simulink model "k1visbs"  (Simulink 8.6)
settings: Solver=ode45  StartTime=0.0  StopTime=10.0  RelTol=1e-3
libraries: cdsEpicsOut x10, cdsBit2Word x10, cdsFilt x8, cdsEpicsBinIn x5, cdsWord2Bit x5, cdsCDI64 x5, cdsCDO64 x5, dac x2, cdsAdcx0 x1, cdsAdcx1 x1, TYPEB_MASTER x1, cdsIPCx x1
(part 1 of 2)
settings Model: Creator=controls  LastModifiedBy=controls
settings DataIOCC: SignalLoggingSaveFormat=Dataset
settings OptimizationCC: ExpressionDepthLimit=128
settings DebuggingCC: UnderspecifiedInitializationDetection=Simplified  MergeDetectMultiDrivingBlocksExec=error  SolverPrmCheckMsg=none  FcnCallInpInsideContextMsg=EnableAllAsError  StateNameClashWarn=none
settings GRTTargetCC: CombineOutputUpdateFcns=on  GRTInterface=off

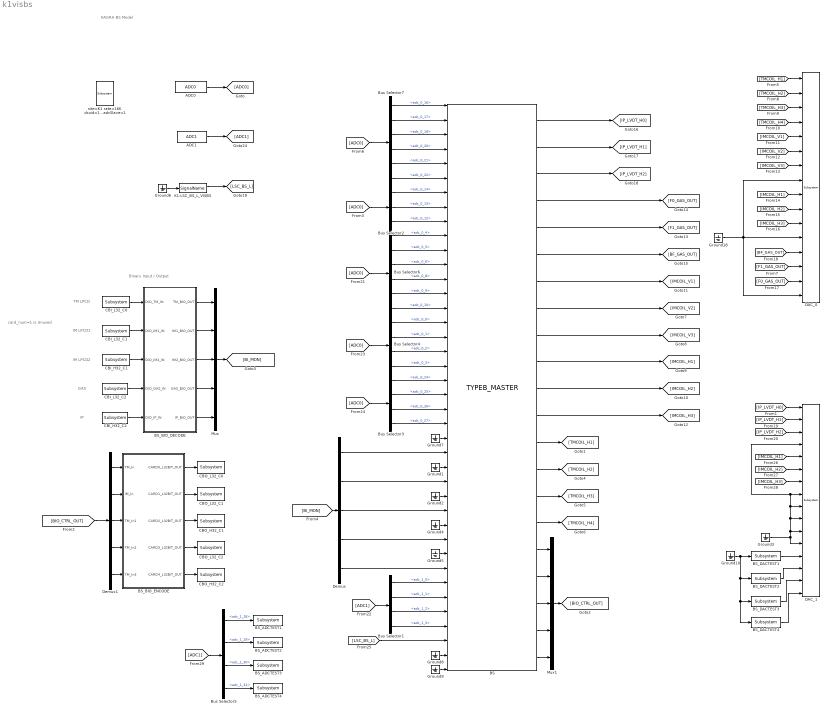
== system k1visbs ==
  note: TM LPCD
  note: KAGRA BS Model
  note: Binary Input / Output
  note: card_num=1 is Unused
  note: IM LPCD1
  note: IM LPCD2
  note: GAS
  note: IP
  ADC0 : cdsAdcx0/ADC0  Tag=cdsAdc  Description=|
      | type-GSC_16AI64SSA
      | card_num=0
      settings: AttributesFormatString=%<Description>\n%<Tag>
  ADC1 : cdsAdcx1/ADC1  Tag=cdsAdc  Description=|
      | type-GSC_16AI64SSA
      | card_num=1
      settings: AttributesFormatString=%<Description>\n%<Tag>
  BS : TYPEB_MASTER/TYPEB_MASTER
  BS_ADCTEST1 : cdsFilt/Subsystem  Tag=cdsFilt  Description=|
      | Purpose:                                                                                                                                                                                                                                  
      | Standard CDS IIR filter module.                                                                                                                                                                                                           
      |                                                                                                                                                                                                                                           
      | Operation:                                                                                                                                                                                                                                
      | Consists of 10 second order section IIR filters, plus a ramped gain stage. In FE code, also provides pre-defined test points and excitation channel inputs. The filter coefficients are defined in the LIGO system using the 'foton' tool.
      |                                                                                                                                                                                                                                           
      | Usage:                                                                                                                                                                                                                                    
      | Name the part with the desired filter module name.
      settings: AttributesFormatString=%<Tag>
  BS_ADCTEST2 : cdsFilt/Subsystem  Tag=cdsFilt  Description=|
      | Purpose:                                                                                                                                                                                                                                  
      | Standard CDS IIR filter module.                                                                                                                                                                                                           
      |                                                                                                                                                                                                                                           
      | Operation:                                                                                                                                                                                                                                
      | Consists of 10 second order section IIR filters, plus a ramped gain stage. In FE code, also provides pre-defined test points and excitation channel inputs. The filter coefficients are defined in the LIGO system using the 'foton' tool.
      |                                                                                                                                                                                                                                           
      | Usage:                                                                                                                                                                                                                                    
      | Name the part with the desired filter module name.
      settings: AttributesFormatString=%<Tag>
  BS_ADCTEST3 : cdsFilt/Subsystem  Tag=cdsFilt  Description=|
      | Purpose:                                                                                                                                                                                                                                  
      | Standard CDS IIR filter module.                                                                                                                                                                                                           
      |                                                                                                                                                                                                                                           
      | Operation:                                                                                                                                                                                                                                
      | Consists of 10 second order section IIR filters, plus a ramped gain stage. In FE code, also provides pre-defined test points and excitation channel inputs. The filter coefficients are defined in the LIGO system using the 'foton' tool.
      |                                                                                                                                                                                                                                           
      | Usage:                                                                                                                                                                                                                                    
      | Name the part with the desired filter module name.
      settings: AttributesFormatString=%<Tag>
  BS_ADCTEST4 : cdsFilt/Subsystem  Tag=cdsFilt  Description=|
      | Purpose:                                                                                                                                                                                                                                  
      | Standard CDS IIR filter module.                                                                                                                                                                                                           
      |                                                                                                                                                                                                                                           
      | Operation:                                                                                                                                                                                                                                
      | Consists of 10 second order section IIR filters, plus a ramped gain stage. In FE code, also provides pre-defined test points and excitation channel inputs. The filter coefficients are defined in the LIGO system using the 'foton' tool.
      |                                                                                                                                                                                                                                           
      | Usage:                                                                                                                                                                                                                                    
      | Name the part with the desired filter module name.
      settings: AttributesFormatString=%<Tag>
  BS_BIO_DECODE : Subsystem
  BS_BIO_ENCODE : Subsystem
  BS_DACTEST1 : cdsFilt/Subsystem  Tag=cdsFilt  Description=|
      | Purpose:                                                                                                                                                                                                                                  
      | Standard CDS IIR filter module.                                                                                                                                                                                                           
      |                                                                                                                                                                                                                                           
      | Operation:                                                                                                                                                                                                                                
      | Consists of 10 second order section IIR filters, plus a ramped gain stage. In FE code, also provides pre-defined test points and excitation channel inputs. The filter coefficients are defined in the LIGO system using the 'foton' tool.
      |                                                                                                                                                                                                                                           
      | Usage:                                                                                                                                                                                                                                    
      | Name the part with the desired filter module name.
      settings: AttributesFormatString=%<Tag>
  BS_DACTEST2 : cdsFilt/Subsystem  Tag=cdsFilt  Description=|
      | Purpose:                                                                                                                                                                                                                                  
      | Standard CDS IIR filter module.                                                                                                                                                                                                           
      |                                                                                                                                                                                                                                           
      | Operation:                                                                                                                                                                                                                                
      | Consists of 10 second order section IIR filters, plus a ramped gain stage. In FE code, also provides pre-defined test points and excitation channel inputs. The filter coefficients are defined in the LIGO system using the 'foton' tool.
      |                                                                                                                                                                                                                                           
      | Usage:                                                                                                                                                                                                                                    
      | Name the part with the desired filter module name.
      settings: AttributesFormatString=%<Tag>
  BS_DACTEST3 : cdsFilt/Subsystem  Tag=cdsFilt  Description=|
      | Purpose:                                                                                                                                                                                                                                  
      | Standard CDS IIR filter module.                                                                                                                                                                                                           
      |                                                                                                                                                                                                                                           
      | Operation:                                                                                                                                                                                                                                
      | Consists of 10 second order section IIR filters, plus a ramped gain stage. In FE code, also provides pre-defined test points and excitation channel inputs. The filter coefficients are defined in the LIGO system using the 'foton' tool.
      |                                                                                                                                                                                                                                           
      | Usage:                                                                                                                                                                                                                                    
      | Name the part with the desired filter module name.
      settings: AttributesFormatString=%<Tag>
  BS_DACTEST4 : cdsFilt/Subsystem  Tag=cdsFilt  Description=|
      | Purpose:                                                                                                                                                                                                                                  
      | Standard CDS IIR filter module.                                                                                                                                                                                                           
      |                                                                                                                                                                                                                                           
      | Operation:                                                                                                                                                                                                                                
      | Consists of 10 second order section IIR filters, plus a ramped gain stage. In FE code, also provides pre-defined test points and excitation channel inputs. The filter coefficients are defined in the LIGO system using the 'foton' tool.
      |                                                                                                                                                                                                                                           
      | Usage:                                                                                                                                                                                                                                    
      | Name the part with the desired filter module name.
      settings: AttributesFormatString=%<Tag>
  Bus Selector1 : BusSelector  Description=ADC Selector  OutputSignals=adc_1_0,adc_1_1,adc_1_2,adc_1_3
      settings: AttributesFormatString=%<Description>
  Bus Selector2 : BusSelector  Description=ADC Selector  OutputSignals=adc_0_14,adc_0_13,adc_0_12
      settings: AttributesFormatString=%<Description>
  Bus Selector3 : BusSelector  Description=ADC Selector  OutputSignals=adc_0_24,adc_0_25,adc_0_26,adc_0_27
      settings: AttributesFormatString=%<Description>
  Bus Selector4 : BusSelector  Description=ADC Selector  OutputSignals=adc_0_0,adc_0_1,adc_0_2,adc_0_3
      settings: AttributesFormatString=%<Description>
  Bus Selector5 : BusSelector  Description=ADC Selector  OutputSignals=adc_1_28,adc_1_29,adc_1_30,adc_1_31
      settings: AttributesFormatString=%<Description>
  Bus Selector6 : BusSelector  Description=ADC Selector  OutputSignals=adc_0_4,adc_0_5,adc_0_6,adc_0_8,adc_0_9,adc_0_10
      settings: AttributesFormatString=%<Description>
  Bus Selector7 : BusSelector  Description=ADC Selector  OutputSignals=adc_0_16,adc_0_17,adc_0_18,adc_0_20,adc_0_21,adc_0_22
      settings: AttributesFormatString=%<Description>
  CBI_H32_C1 : cdsCDI64/Subsystem  Tag=cdsCDI64  Description=card_num=3
      settings: AttributesFormatString=%<Tag>\n%<Description>
  CBI_H32_C2 : cdsCDI64/Subsystem  Tag=cdsCDI64  Description=card_num=5
      settings: AttributesFormatString=%<Tag>\n%<Description>
  CBI_L32_C0 : cdsCDI64/Subsystem  Tag=cdsCDI64  Description=card_num=0
      settings: AttributesFormatString=%<Tag>\n%<Description>
  CBI_L32_C1 : cdsCDI64/Subsystem  Tag=cdsCDI64  Description=card_num=2
      settings: AttributesFormatString=%<Tag>\n%<Description>
  CBI_L32_C2 : cdsCDI64/Subsystem  Tag=cdsCDI64  Description=card_num=4
      settings: AttributesFormatString=%<Tag>\n%<Description>
  CBO_H32_C1 : cdsCDO64/Subsystem  Tag=cdsCDO64  Description=card_num=3
      settings: AttributesFormatString=%<Tag>\n%<Description>
  CBO_H32_C2 : cdsCDO64/Subsystem  Tag=cdsCDO64  Description=card_num=5
      settings: AttributesFormatString=%<Tag>\n%<Description>
  CBO_L32_C0 : cdsCDO64/Subsystem  Tag=cdsCDO64  Description=card_num=0
      settings: AttributesFormatString=%<Tag>\n%<Description>
  CBO_L32_C1 : cdsCDO64/Subsystem  Tag=cdsCDO64  Description=card_num=2
      settings: AttributesFormatString=%<Tag>\n%<Description>
  CBO_L32_C2 : cdsCDO64/Subsystem  Tag=cdsCDO64  Description=card_num=4
      settings: AttributesFormatString=%<Tag>\n%<Description>
  DAC_0 : dac/Subsystem  Description=|
      | type=GSC_16AO16,
      | card_num=0
      settings: AttributesFormatString=%<Description>
  DAC_1 : dac/Subsystem  Description=|
      | type=GSC_16AO16,
      | card_num=1
      settings: AttributesFormatString=%<Description>
  Demux : Demux  Outputs=5
  Demux1 : Demux  Outputs=5
  Ground{1..10,18} (11 alike) : Ground
  K1:LSC_BS_L_VISBS : cdsIPCx/SignalName  Tag=cdsIPCx_PCIE  Description=Inter-Process Communication via PCI Express network.
      settings: AttributesFormatString=%<Tag>
  Mux : Mux  Inputs=5
  Mux1 : Mux  Inputs=5
  site=K1 rate=16K dcuid=1096 host=k1bs specific_cpu=4 adcSlave=1 : cdsParameters/Subsystem  Tag=cdsParameters  Description=|
      | Purpose:                                                                                                                                                                                                                                
      | Provide system parameters to the FE code generator to properly configure the generated EPICS names, rep rate of the FE controller, and the Data Acquisition node ID for proper storage of data from this FE controller.                 
      |                                                                                                                                                                                                                                         
      | Useage:                                                                                                                                                                                                                                 
      | The part NAME field is used to identify the FE parameters. It must be of the form:                                                                                                                                                      
      | site=                                                                                                                                                                                                                                   
      | rate=                                                                                                                                                                                                                                   
      | dcuid=                                                                                                                                                                                                                                  
      |                                                                                                                                                                                                                                         
      | Where:                                                                                                                                                                                                                                  
      | site= argument may be H1, H2, L1, M1, G1, either as a single argument or multiple, for example site=H1,H2. These are the only names allowed. These will become the first two characters of all EPICS and signal names (for example G1:).
      |                                                                                                                                                                                                                                         
      | rate= may be 2K, 16K, 32K, or 64K                                                                                                                                                                                                       
      |                                                                                                                                                                                                                                         
      | dcuid= is site specific ie it must be unique at each site.
      settings: AttributesFormatString=%<Tag>
  wires:
  BS/4 -> [F0_GAS_OUT]
  BS/5 -> [F1_GAS_OUT]
  BS/6 -> [BF_GAS_OUT]
  ADC0/1 -> [ADC0]
  [ADC0] -> Bus Selector6/1
  [ADC0] -> Bus Selector3/1
  [ADC0] -> Bus Selector7/1
  BS/16 -> [TMCOIL_H4]
  BS/15 -> [TMCOIL_H3]
  BS/14 -> [TMCOIL_H2]
  BS/13 -> [TMCOIL_H1]
  BS/7 -> [IMCOIL_V1]
  BS/8 -> [IMCOIL_V2]
  BS/9 -> [IMCOIL_V3]
  BS/10 -> [IMCOIL_H1]
  BS/11 -> [IMCOIL_H2]
  BS/12 -> [IMCOIL_H3]
  ADC1/1 -> [ADC1]
  Ground3/1 -> DAC_1/12, DAC_1/4, DAC_1/8, DAC_1/9, DAC_1/10, DAC_1/11
  [ADC0] -> Bus Selector2/1
  Bus Selector2/2 -> BS/8  "<adc_0_13>"
  Bus Selector2/3 -> BS/9  "<adc_0_12>"
  Bus Selector7/1 -> BS/1  "<adc_0_16>"
  Bus Selector7/2 -> BS/2  "<adc_0_17>"
  Bus Selector7/3 -> BS/3  "<adc_0_18>"
  Bus Selector7/4 -> BS/4  "<adc_0_20>"
  Bus Selector7/5 -> BS/5  "<adc_0_21>"
  Bus Selector7/6 -> BS/6  "<adc_0_22>"
  Ground7/1 -> BS/24
  BS_BIO_ENCODE/1(CARD0_L32BIT_OUT) -> CBO_L32_C0/1
  BS_BIO_ENCODE/3(CARD2_L32BIT_OUT) -> CBO_H32_C1/1
  BS_BIO_ENCODE/2(CARD1_L32BIT_OUT) -> CBO_L32_C1/1
  BS_BIO_ENCODE/4(CARD3_L32BIT_OUT) -> CBO_L32_C2/1
  CBI_L32_C0/1 -> BS_BIO_DECODE/1(DIO_TM_IN)
  CBI_L32_C1/1 -> BS_BIO_DECODE/2(DIO_IM1_IN)
  CBI_H32_C1/1 -> BS_BIO_DECODE/3(DIO_IM2_IN)
  CBI_L32_C2/1 -> BS_BIO_DECODE/4(DIO_GAS_IN)
  BS/21 -> Mux1/5
  BS_BIO_DECODE/2(IM1_BIO_OUT) -> Mux/2
  BS_BIO_DECODE/3(IM2_BIO_OUT) -> Mux/3
  BS_BIO_DECODE/4(GAS_BIO_OUT) -> Mux/4
  BS_BIO_DECODE/5(IP_BIO_OUT) -> Mux/5
  BS_BIO_DECODE/1(TM_BIO_OUT) -> Mux/1
  Mux/1 -> [BI_MON]
  Demux/1 -> BS/25
  [BI_MON] -> Demux/1
  Demux/4 -> BS/31
  Demux/3 -> BS/29
  Demux/2 -> BS/27
  Ground1/1 -> BS/26
  Ground2/1 -> BS/28
  Ground4/1 -> BS/30
  Mux1/1 -> [BIO_CTRL_OUT]
  BS/17 -> Mux1/1
  BS/18 -> Mux1/2
  BS/19 -> Mux1/3
  BS/20 -> Mux1/4
  Demux1/2 -> BS_BIO_ENCODE/2(IM_In)
  Demux1/3 -> BS_BIO_ENCODE/3(TM_In1)
  Demux1/4 -> BS_BIO_ENCODE/4(TM_In2)
  Demux1/1 -> BS_BIO_ENCODE/1(TM_In)
  [BIO_CTRL_OUT] -> Demux1/1
  CBI_H32_C2/1 -> BS_BIO_DECODE/5(DIO_IP_IN)
  BS_BIO_ENCODE/5(CARD4_L32BIT_OUT) -> CBO_H32_C2/1
  Demux1/5 -> BS_BIO_ENCODE/5(TM_In3)
  Ground18/1 -> DAC_0/8, DAC_0/16, DAC_0/12
  [F1_GAS_OUT] -> DAC_0/14
  [F0_GAS_OUT] -> DAC_0/15
  [BF_GAS_OUT] -> DAC_0/13
  BS/2 -> [IP_LVDT_H1]
  BS/1 -> [IP_LVDT_H0]
  BS/3 -> [IP_LVDT_H2]
  [IP_LVDT_H0] -> DAC_1/1
  [IP_LVDT_H1] -> DAC_1/2
  [IP_LVDT_H2] -> DAC_1/3
  Bus Selector2/1 -> BS/7  "<adc_0_14>"
  [ADC1] -> Bus Selector1/1
  Bus Selector3/1 -> BS/20  "<adc_0_24>"
  Bus Selector3/2 -> BS/21  "<adc_0_25>"
  Bus Selector3/3 -> BS/22  "<adc_0_26>"
  Bus Selector3/4 -> BS/23  "<adc_0_27>"
  [ADC0] -> Bus Selector4/1
  Bus Selector6/1 -> BS/10  "<adc_0_4>"
  Bus Selector6/2 -> BS/11  "<adc_0_5>"
  Bus Selector6/3 -> BS/12  "<adc_0_6>"
  Bus Selector4/1 -> BS/16  "<adc_0_0>"
  Bus Selector4/2 -> BS/17  "<adc_0_1>"
  Bus Selector4/3 -> BS/18  "<adc_0_2>"
  Bus Selector4/4 -> BS/19  "<adc_0_3>"
  [TMCOIL_H2] -> DAC_0/2
  [TMCOIL_H3] -> DAC_0/3
  [TMCOIL_H1] -> DAC_0/1
  [TMCOIL_H4] -> DAC_0/4
  [IMCOIL_V1] -> DAC_0/5
  [IMCOIL_V2] -> DAC_0/6
  [IMCOIL_V3] -> DAC_0/7
  Bus Selector6/4 -> BS/13  "<adc_0_8>"
  Bus Selector6/5 -> BS/14  "<adc_0_9>"
  Bus Selector6/6 -> BS/15  "<adc_0_10>"
  [IMCOIL_H3] -> DAC_0/11
  [IMCOIL_H2] -> DAC_0/10
  [IMCOIL_H1] -> DAC_0/9
  Bus Selector1/1 -> BS/34  "<adc_1_0>"
  Bus Selector1/2 -> BS/35  "<adc_1_1>"
  Bus Selector1/3 -> BS/36  "<adc_1_2>"
  Bus Selector1/4 -> BS/37  "<adc_1_3>"
  Demux/5 -> BS/33
  Ground5/1 -> BS/32
  Ground6/1 -> K1:LSC_BS_L_VISBS/1
  K1:LSC_BS_L_VISBS/1 -> [LSC_BS_L]
  [LSC_BS_L] -> BS/38
  Ground8/1 -> BS/39
  Ground9/1 -> BS/40
  [IMCOIL_H3] -> DAC_1/7
  [IMCOIL_H2] -> DAC_1/6
  [IMCOIL_H1] -> DAC_1/5
  BS_DACTEST3/1 -> DAC_1/15
  BS_DACTEST4/1 -> DAC_1/16
  BS_DACTEST2/1 -> DAC_1/14
  BS_DACTEST1/1 -> DAC_1/13
  Ground10/1 -> BS_DACTEST4/1, BS_DACTEST3/1, BS_DACTEST2/1, BS_DACTEST1/1
  [ADC1] -> Bus Selector5/1
  Bus Selector5/1 -> BS_ADCTEST1/1  "<adc_1_28>"
  Bus Selector5/2 -> BS_ADCTEST2/1  "<adc_1_29>"
  Bus Selector5/3 -> BS_ADCTEST3/1  "<adc_1_30>"
  Bus Selector5/4 -> BS_ADCTEST4/1  "<adc_1_31>"

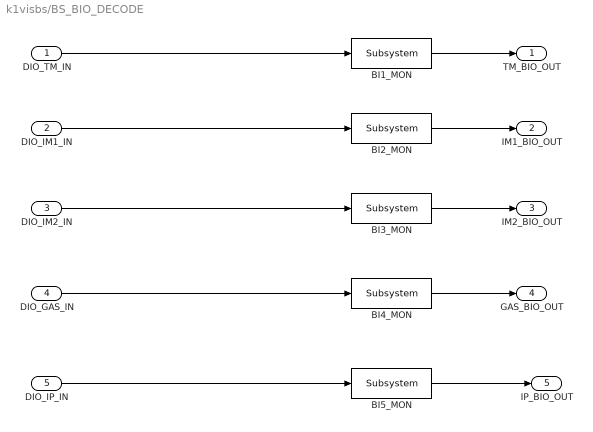
== system k1visbs/BS_BIO_DECODE ==
  DIO_TM_IN : Inport
  DIO_IM1_IN : Inport  Port=2
  DIO_IM2_IN : Inport  Port=3
  DIO_GAS_IN : Inport  Port=4
  DIO_IP_IN : Inport  Port=5
  BI1_MON : cdsEpicsOut/Subsystem  Tag=cdsEpicsOutput  Description=|
      | Purpose:                                          
      | Output a FE signal to an EPICS channel.           
      |                                                   
      | Operation:                                        
      | Takes input value and passes it to EPICS record.  
      |                                                   
      | Usage:                                            
      | Name the part with the desired EPICS rrecord name.
      settings: AttributesFormatString=%<Tag>
  BI2_MON : cdsEpicsOut/Subsystem  Tag=cdsEpicsOutput  Description=|
      | Purpose:                                          
      | Output a FE signal to an EPICS channel.           
      |                                                   
      | Operation:                                        
      | Takes input value and passes it to EPICS record.  
      |                                                   
      | Usage:                                            
      | Name the part with the desired EPICS rrecord name.
      settings: AttributesFormatString=%<Tag>
  BI3_MON : cdsEpicsOut/Subsystem  Tag=cdsEpicsOutput  Description=|
      | Purpose:                                          
      | Output a FE signal to an EPICS channel.           
      |                                                   
      | Operation:                                        
      | Takes input value and passes it to EPICS record.  
      |                                                   
      | Usage:                                            
      | Name the part with the desired EPICS rrecord name.
      settings: AttributesFormatString=%<Tag>
  BI4_MON : cdsEpicsOut/Subsystem  Tag=cdsEpicsOutput  Description=|
      | Purpose:                                          
      | Output a FE signal to an EPICS channel.           
      |                                                   
      | Operation:                                        
      | Takes input value and passes it to EPICS record.  
      |                                                   
      | Usage:                                            
      | Name the part with the desired EPICS rrecord name.
      settings: AttributesFormatString=%<Tag>
  BI5_MON : cdsEpicsOut/Subsystem  Tag=cdsEpicsOutput  Description=|
      | Purpose:                                          
      | Output a FE signal to an EPICS channel.           
      |                                                   
      | Operation:                                        
      | Takes input value and passes it to EPICS record.  
      |                                                   
      | Usage:                                            
      | Name the part with the desired EPICS rrecord name.
      settings: AttributesFormatString=%<Tag>
  TM_BIO_OUT : Outport
  IM1_BIO_OUT : Outport  Port=2
  IM2_BIO_OUT : Outport  Port=3
  GAS_BIO_OUT : Outport  Port=4
  IP_BIO_OUT : Outport  Port=5
  wires:
  DIO_IM1_IN/1 -> BI2_MON/1
  DIO_TM_IN/1 -> BI1_MON/1
  DIO_IM2_IN/1 -> BI3_MON/1
  DIO_GAS_IN/1 -> BI4_MON/1
  BI1_MON/1 -> TM_BIO_OUT/1
  DIO_IP_IN/1 -> BI5_MON/1
  BI2_MON/1 -> IM1_BIO_OUT/1
  BI3_MON/1 -> IM2_BIO_OUT/1
  BI4_MON/1 -> GAS_BIO_OUT/1
  BI5_MON/1 -> IP_BIO_OUT/1

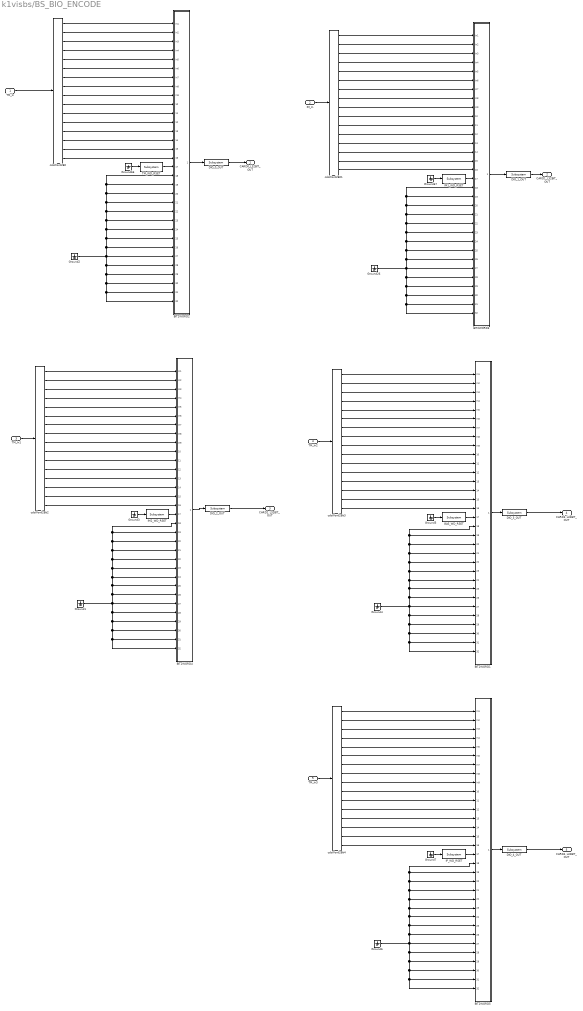
== system k1visbs/BS_BIO_ENCODE ==
  TM_In : Inport
  IM_In : Inport  Port=2
  TM_In1 : Inport  Port=3
  TM_In2 : Inport  Port=4
  TM_In3 : Inport  Port=5
  BIT2WORD1 : Subsystem
  BIT2WORD2 : Subsystem
  BIT2WORD3 : Subsystem
  BIT2WORD4 : Subsystem
  BIT2WORD5 : Subsystem
  DIO_0_OUT : cdsEpicsOut/Subsystem  Tag=cdsEpicsOutput  Description=|
      | Purpose:                                          
      | Output a FE signal to an EPICS channel.           
      |                                                   
      | Operation:                                        
      | Takes input value and passes it to EPICS record.  
      |                                                   
      | Usage:                                            
      | Name the part with the desired EPICS rrecord name.
      settings: AttributesFormatString=%<Tag>
  DIO_1_OUT : cdsEpicsOut/Subsystem  Tag=cdsEpicsOutput  Description=|
      | Purpose:                                          
      | Output a FE signal to an EPICS channel.           
      |                                                   
      | Operation:                                        
      | Takes input value and passes it to EPICS record.  
      |                                                   
      | Usage:                                            
      | Name the part with the desired EPICS rrecord name.
      settings: AttributesFormatString=%<Tag>
  DIO_2_OUT : cdsEpicsOut/Subsystem  Tag=cdsEpicsOutput  Description=|
      | Purpose:                                          
      | Output a FE signal to an EPICS channel.           
      |                                                   
      | Operation:                                        
      | Takes input value and passes it to EPICS record.  
      |                                                   
      | Usage:                                            
      | Name the part with the desired EPICS rrecord name.
      settings: AttributesFormatString=%<Tag>
  DIO_3_OUT : cdsEpicsOut/Subsystem  Tag=cdsEpicsOutput  Description=|
      | Purpose:                                          
      | Output a FE signal to an EPICS channel.           
      |                                                   
      | Operation:                                        
      | Takes input value and passes it to EPICS record.  
      |                                                   
      | Usage:                                            
      | Name the part with the desired EPICS rrecord name.
      settings: AttributesFormatString=%<Tag>
  DIO_4_OUT : cdsEpicsOut/Subsystem  Tag=cdsEpicsOutput  Description=|
      | Purpose:                                          
      | Output a FE signal to an EPICS channel.           
      |                                                   
      | Operation:                                        
      | Takes input value and passes it to EPICS record.  
      |                                                   
      | Usage:                                            
      | Name the part with the desired EPICS rrecord name.
      settings: AttributesFormatString=%<Tag>
  GAS_WD_RSET : cdsEpicsBinIn/Subsystem  Tag=cdsEpicsBinIn  Description=|
      | Purpose:                                                                            
      | Create an EPICS binary (0 or 1) input channel to the FE realtime controls.          
      |                                                                                     
      | Operation:                                                                          
      | Outputs value from an EPICS ai record. Value is binary input (bi Epics record type).
      |                                                                                     
      | Usage:                                                                              
      | Name the part with the desired EPICS channel name.
      settings: AttributesFormatString=%<Tag>
  Ground{1..7,26,66..67} (10 alike) : Ground
  IM1_WD_RSET : cdsEpicsBinIn/Subsystem  Tag=cdsEpicsBinIn  Description=|
      | Purpose:                                                                            
      | Create an EPICS binary (0 or 1) input channel to the FE realtime controls.          
      |                                                                                     
      | Operation:                                                                          
      | Outputs value from an EPICS ai record. Value is binary input (bi Epics record type).
      |                                                                                     
      | Usage:                                                                              
      | Name the part with the desired EPICS channel name.
      settings: AttributesFormatString=%<Tag>
  IM2_WD_RSET : cdsEpicsBinIn/Subsystem  Tag=cdsEpicsBinIn  Description=|
      | Purpose:                                                                            
      | Create an EPICS binary (0 or 1) input channel to the FE realtime controls.          
      |                                                                                     
      | Operation:                                                                          
      | Outputs value from an EPICS ai record. Value is binary input (bi Epics record type).
      |                                                                                     
      | Usage:                                                                              
      | Name the part with the desired EPICS channel name.
      settings: AttributesFormatString=%<Tag>
  IP_WD_RSET : cdsEpicsBinIn/Subsystem  Tag=cdsEpicsBinIn  Description=|
      | Purpose:                                                                            
      | Create an EPICS binary (0 or 1) input channel to the FE realtime controls.          
      |                                                                                     
      | Operation:                                                                          
      | Outputs value from an EPICS ai record. Value is binary input (bi Epics record type).
      |                                                                                     
      | Usage:                                                                              
      | Name the part with the desired EPICS channel name.
      settings: AttributesFormatString=%<Tag>
  TM_WD_RSET : cdsEpicsBinIn/Subsystem  Tag=cdsEpicsBinIn  Description=|
      | Purpose:                                                                            
      | Create an EPICS binary (0 or 1) input channel to the FE realtime controls.          
      |                                                                                     
      | Operation:                                                                          
      | Outputs value from an EPICS ai record. Value is binary input (bi Epics record type).
      |                                                                                     
      | Usage:                                                                              
      | Name the part with the desired EPICS channel name.
      settings: AttributesFormatString=%<Tag>
  cdsWord2Bit{,1..4} (5 alike) : cdsWord2Bit/cdsWord2Bit  Tag=cdsWord2Bit  Description=Generate 16 0/1 outputs from single 16-bit integer input
      settings: AttributesFormatString=cdsWord2Bit
  CARD0_L32BIT_OUT : Outport
  CARD1_L32BIT_OUT : Outport  Port=2
  CARD2_L32BIT_OUT : Outport  Port=3
  CARD3_L32BIT_OUT : Outport  Port=4
  CARD4_L32BIT_OUT : Outport  Port=5
  wires:
  Ground2/1 -> BIT2WORD2/20(In20), BIT2WORD2/18(In18), BIT2WORD2/19(In19), BIT2WORD2/21(In21), BIT2WORD2/22(In22), BIT2WORD2/23(In23), BIT2WORD2/24(In24), BIT2WORD2/25(In25), BIT2WORD2/26(In26), BIT2WORD2/28(In28), BIT2WORD2/31(In31), BIT2WORD2/32(In32), BIT2WORD2/30(In30), BIT2WORD2/29(In29), BIT2WORD2/27(In27)
  TM_In/1 -> cdsWord2Bit/1
  cdsWord2Bit/4 -> BIT2WORD2/4(In4)
  cdsWord2Bit/5 -> BIT2WORD2/5(In5)
  cdsWord2Bit/3 -> BIT2WORD2/3(In3)
  cdsWord2Bit/2 -> BIT2WORD2/2(In2)
  cdsWord2Bit/6 -> BIT2WORD2/6(In6)
  cdsWord2Bit/1 -> BIT2WORD2/1(In1)
  cdsWord2Bit/7 -> BIT2WORD2/7(In7)
  cdsWord2Bit/8 -> BIT2WORD2/8(In8)
  cdsWord2Bit/9 -> BIT2WORD2/9(In9)
  cdsWord2Bit/10 -> BIT2WORD2/10(In10)
  cdsWord2Bit/11 -> BIT2WORD2/11(In11)
  Ground26/1 -> BIT2WORD3/20(In20), BIT2WORD3/18(In18), BIT2WORD3/19(In19), BIT2WORD3/21(In21), BIT2WORD3/22(In22), BIT2WORD3/23(In23), BIT2WORD3/24(In24), BIT2WORD3/25(In25), BIT2WORD3/26(In26), BIT2WORD3/28(In28), BIT2WORD3/31(In31), BIT2WORD3/32(In32), BIT2WORD3/30(In30), BIT2WORD3/29(In29), BIT2WORD3/27(In27)
  IM_In/1 -> cdsWord2Bit1/1
  cdsWord2Bit1/4 -> BIT2WORD3/4(In4)
  cdsWord2Bit1/5 -> BIT2WORD3/5(In5)
  cdsWord2Bit1/3 -> BIT2WORD3/3(In3)
  cdsWord2Bit1/2 -> BIT2WORD3/2(In2)
  cdsWord2Bit1/6 -> BIT2WORD3/6(In6)
  cdsWord2Bit1/1 -> BIT2WORD3/1(In1)
  cdsWord2Bit1/7 -> BIT2WORD3/7(In7)
  cdsWord2Bit1/8 -> BIT2WORD3/8(In8)
  cdsWord2Bit1/9 -> BIT2WORD3/9(In9)
  cdsWord2Bit1/10 -> BIT2WORD3/10(In10)
  cdsWord2Bit1/11 -> BIT2WORD3/11(In11)
  Ground66/1 -> TM_WD_RSET/1
  Ground67/1 -> IM1_WD_RSET/1
  TM_WD_RSET/1 -> BIT2WORD2/17(In17)
  IM1_WD_RSET/1 -> BIT2WORD3/17(In17)
  DIO_0_OUT/1 -> CARD0_L32BIT_OUT/1
  DIO_2_OUT/1 -> CARD2_L32BIT_OUT/1
  BIT2WORD2/1(Out1) -> DIO_0_OUT/1
  BIT2WORD3/1(Out1) -> DIO_1_OUT/1
  DIO_1_OUT/1 -> CARD1_L32BIT_OUT/1
  BIT2WORD4/1(Out1) -> DIO_2_OUT/1
  BIT2WORD1/1(Out1) -> DIO_3_OUT/1
  DIO_3_OUT/1 -> CARD3_L32BIT_OUT/1
  Ground1/1 -> BIT2WORD4/27(In27), BIT2WORD4/26(In26), BIT2WORD4/25(In25), BIT2WORD4/24(In24), BIT2WORD4/23(In23), BIT2WORD4/22(In22), BIT2WORD4/21(In21), BIT2WORD4/20(In20), BIT2WORD4/19(In19), BIT2WORD4/18(In18), BIT2WORD4/28(In28), BIT2WORD4/29(In29), BIT2WORD4/30(In30), BIT2WORD4/32(In32), BIT2WORD4/31(In31)
  TM_In1/1 -> cdsWord2Bit2/1
  cdsWord2Bit2/4 -> BIT2WORD4/4(In4)
  cdsWord2Bit2/5 -> BIT2WORD4/5(In5)
  cdsWord2Bit2/3 -> BIT2WORD4/3(In3)
  cdsWord2Bit2/2 -> BIT2WORD4/2(In2)
  cdsWord2Bit2/6 -> BIT2WORD4/6(In6)
  cdsWord2Bit2/1 -> BIT2WORD4/1(In1)
  cdsWord2Bit2/7 -> BIT2WORD4/7(In7)
  cdsWord2Bit2/8 -> BIT2WORD4/8(In8)
  cdsWord2Bit2/9 -> BIT2WORD4/9(In9)
  cdsWord2Bit2/10 -> BIT2WORD4/10(In10)
  cdsWord2Bit2/11 -> BIT2WORD4/11(In11)
  Ground3/1 -> IM2_WD_RSET/1
  IM2_WD_RSET/1 -> BIT2WORD4/17(In17)
  Ground4/1 -> BIT2WORD1/27(In27), BIT2WORD1/26(In26), BIT2WORD1/25(In25), BIT2WORD1/24(In24), BIT2WORD1/23(In23), BIT2WORD1/22(In22), BIT2WORD1/21(In21), BIT2WORD1/20(In20), BIT2WORD1/19(In19), BIT2WORD1/18(In18), BIT2WORD1/28(In28), BIT2WORD1/29(In29), BIT2WORD1/30(In30), BIT2WORD1/32(In32), BIT2WORD1/31(In31)
  TM_In2/1 -> cdsWord2Bit3/1
  cdsWord2Bit3/4 -> BIT2WORD1/4(In4)
  cdsWord2Bit3/5 -> BIT2WORD1/5(In5)
  cdsWord2Bit3/3 -> BIT2WORD1/3(In3)
  cdsWord2Bit3/2 -> BIT2WORD1/2(In2)
  cdsWord2Bit3/6 -> BIT2WORD1/6(In6)
  cdsWord2Bit3/1 -> BIT2WORD1/1(In1)
  cdsWord2Bit3/7 -> BIT2WORD1/7(In7)
  cdsWord2Bit3/8 -> BIT2WORD1/8(In8)
  cdsWord2Bit3/9 -> BIT2WORD1/9(In9)
  cdsWord2Bit3/10 -> BIT2WORD1/10(In10)
  cdsWord2Bit3/11 -> BIT2WORD1/11(In11)
  Ground5/1 -> GAS_WD_RSET/1
  GAS_WD_RSET/1 -> BIT2WORD1/17(In17)
  cdsWord2Bit/12 -> BIT2WORD2/12(In12)
  cdsWord2Bit/13 -> BIT2WORD2/13(In13)
  cdsWord2Bit/14 -> BIT2WORD2/14(In14)
  cdsWord2Bit/15 -> BIT2WORD2/15(In15)
  cdsWord2Bit/16 -> BIT2WORD2/16(In16)
  cdsWord2Bit1/12 -> BIT2WORD3/12(In12)
  cdsWord2Bit1/16 -> BIT2WORD3/16(In16)
  cdsWord2Bit1/14 -> BIT2WORD3/14(In14)
  cdsWord2Bit1/15 -> BIT2WORD3/15(In15)
  cdsWord2Bit1/13 -> BIT2WORD3/13(In13)
  cdsWord2Bit3/13 -> BIT2WORD1/13(In13)
  cdsWord2Bit3/14 -> BIT2WORD1/14(In14)
  cdsWord2Bit3/15 -> BIT2WORD1/15(In15)
  cdsWord2Bit3/16 -> BIT2WORD1/16(In16)
  cdsWord2Bit3/12 -> BIT2WORD1/12(In12)
  cdsWord2Bit2/13 -> BIT2WORD4/13(In13)
  cdsWord2Bit2/15 -> BIT2WORD4/15(In15)
  cdsWord2Bit2/14 -> BIT2WORD4/14(In14)
  cdsWord2Bit2/12 -> BIT2WORD4/12(In12)
  cdsWord2Bit2/16 -> BIT2WORD4/16(In16)
  BIT2WORD5/1(Out1) -> DIO_4_OUT/1
  DIO_4_OUT/1 -> CARD4_L32BIT_OUT/1
  Ground6/1 -> BIT2WORD5/27(In27), BIT2WORD5/26(In26), BIT2WORD5/25(In25), BIT2WORD5/24(In24), BIT2WORD5/23(In23), BIT2WORD5/22(In22), BIT2WORD5/21(In21), BIT2WORD5/20(In20), BIT2WORD5/19(In19), BIT2WORD5/18(In18), BIT2WORD5/28(In28), BIT2WORD5/29(In29), BIT2WORD5/30(In30), BIT2WORD5/32(In32), BIT2WORD5/31(In31)
  TM_In3/1 -> cdsWord2Bit4/1
  cdsWord2Bit4/4 -> BIT2WORD5/4(In4)
  cdsWord2Bit4/5 -> BIT2WORD5/5(In5)
  cdsWord2Bit4/3 -> BIT2WORD5/3(In3)
  cdsWord2Bit4/2 -> BIT2WORD5/2(In2)
  cdsWord2Bit4/6 -> BIT2WORD5/6(In6)
  cdsWord2Bit4/1 -> BIT2WORD5/1(In1)
  cdsWord2Bit4/7 -> BIT2WORD5/7(In7)
  cdsWord2Bit4/8 -> BIT2WORD5/8(In8)
  cdsWord2Bit4/9 -> BIT2WORD5/9(In9)
  cdsWord2Bit4/10 -> BIT2WORD5/10(In10)
  cdsWord2Bit4/11 -> BIT2WORD5/11(In11)
  Ground7/1 -> IP_WD_RSET/1
  IP_WD_RSET/1 -> BIT2WORD5/17(In17)
  cdsWord2Bit4/13 -> BIT2WORD5/13(In13)
  cdsWord2Bit4/14 -> BIT2WORD5/14(In14)
  cdsWord2Bit4/15 -> BIT2WORD5/15(In15)
  cdsWord2Bit4/16 -> BIT2WORD5/16(In16)
  cdsWord2Bit4/12 -> BIT2WORD5/12(In12)

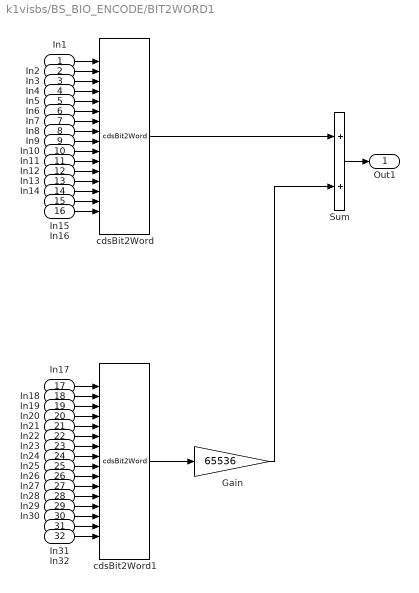
== system k1visbs/BS_BIO_ENCODE/BIT2WORD1 ==
  In1 : Inport
  In2 : Inport  Port=2
  In3 : Inport  Port=3
  In4 : Inport  Port=4
  In5 : Inport  Port=5
  In6 : Inport  Port=6
  In7 : Inport  Port=7
  In8 : Inport  Port=8
  In9 : Inport  Port=9
  In10 : Inport  Port=10
  In11 : Inport  Port=11
  In12 : Inport  Port=12
  In13 : Inport  Port=13
  In14 : Inport  Port=14
  In15 : Inport  Port=15
  In16 : Inport  Port=16
  In17 : Inport  Port=17
  In18 : Inport  Port=18
  In19 : Inport  Port=19
  In20 : Inport  Port=20
  In21 : Inport  Port=21
  In22 : Inport  Port=22
  In23 : Inport  Port=23
  In24 : Inport  Port=24
  In25 : Inport  Port=25
  In26 : Inport  Port=26
  In27 : Inport  Port=27
  In28 : Inport  Port=28
  In29 : Inport  Port=29
  In30 : Inport  Port=30
  In31 : Inport  Port=31
  In32 : Inport  Port=32
  Gain : Gain  Gain=65536
  Sum : Sum
  cdsBit2Word : cdsBit2Word/cdsBit2Word  Tag=cdsBit2Word  Description=Forms single 16 bit integer from 16 0/1 inputs.
      settings: AttributesFormatString=%<Tag>
  cdsBit2Word1 : cdsBit2Word/cdsBit2Word  Tag=cdsBit2Word  Description=Forms single 16 bit integer from 16 0/1 inputs.
      settings: AttributesFormatString=%<Tag>
  Out1 : Outport
  wires:
  Gain/1 -> Sum/2
  cdsBit2Word1/1 -> Gain/1
  cdsBit2Word/1 -> Sum/1
  In1/1 -> cdsBit2Word/1
  In2/1 -> cdsBit2Word/2
  In3/1 -> cdsBit2Word/3
  In4/1 -> cdsBit2Word/4
  In5/1 -> cdsBit2Word/5
  In6/1 -> cdsBit2Word/6
  In7/1 -> cdsBit2Word/7
  In8/1 -> cdsBit2Word/8
  In9/1 -> cdsBit2Word/9
  In10/1 -> cdsBit2Word/10
  Sum/1 -> Out1/1
  In11/1 -> cdsBit2Word/11
  In12/1 -> cdsBit2Word/12
  In13/1 -> cdsBit2Word/13
  In14/1 -> cdsBit2Word/14
  In15/1 -> cdsBit2Word/15
  In16/1 -> cdsBit2Word/16
  In17/1 -> cdsBit2Word1/1
  In18/1 -> cdsBit2Word1/2
  In19/1 -> cdsBit2Word1/3
  In20/1 -> cdsBit2Word1/4
  In21/1 -> cdsBit2Word1/5
  In22/1 -> cdsBit2Word1/6
  In23/1 -> cdsBit2Word1/7
  In24/1 -> cdsBit2Word1/8
  In25/1 -> cdsBit2Word1/9
  In26/1 -> cdsBit2Word1/10
  In27/1 -> cdsBit2Word1/11
  In28/1 -> cdsBit2Word1/12
  In29/1 -> cdsBit2Word1/13
  In30/1 -> cdsBit2Word1/14
  In31/1 -> cdsBit2Word1/15
  In32/1 -> cdsBit2Word1/16

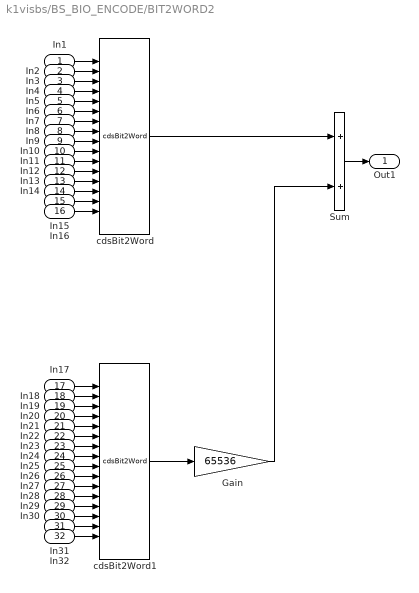
== system k1visbs/BS_BIO_ENCODE/BIT2WORD2 ==
  In1 : Inport
  In2 : Inport  Port=2
  In3 : Inport  Port=3
  In4 : Inport  Port=4
  In5 : Inport  Port=5
  In6 : Inport  Port=6
  In7 : Inport  Port=7
  In8 : Inport  Port=8
  In9 : Inport  Port=9
  In10 : Inport  Port=10
  In11 : Inport  Port=11
  In12 : Inport  Port=12
  In13 : Inport  Port=13
  In14 : Inport  Port=14
  In15 : Inport  Port=15
  In16 : Inport  Port=16
  In17 : Inport  Port=17
  In18 : Inport  Port=18
  In19 : Inport  Port=19
  In20 : Inport  Port=20
  In21 : Inport  Port=21
  In22 : Inport  Port=22
  In23 : Inport  Port=23
  In24 : Inport  Port=24
  In25 : Inport  Port=25
  In26 : Inport  Port=26
  In27 : Inport  Port=27
  In28 : Inport  Port=28
  In29 : Inport  Port=29
  In30 : Inport  Port=30
  In31 : Inport  Port=31
  In32 : Inport  Port=32
  Gain : Gain  Gain=65536
  Sum : Sum
  cdsBit2Word : cdsBit2Word/cdsBit2Word  Tag=cdsBit2Word  Description=Forms single 16 bit integer from 16 0/1 inputs.
      settings: AttributesFormatString=%<Tag>
  cdsBit2Word1 : cdsBit2Word/cdsBit2Word  Tag=cdsBit2Word  Description=Forms single 16 bit integer from 16 0/1 inputs.
      settings: AttributesFormatString=%<Tag>
  Out1 : Outport
  wires:
  Gain/1 -> Sum/2
  cdsBit2Word1/1 -> Gain/1
  cdsBit2Word/1 -> Sum/1
  In1/1 -> cdsBit2Word/1
  In2/1 -> cdsBit2Word/2
  In3/1 -> cdsBit2Word/3
  In4/1 -> cdsBit2Word/4
  In5/1 -> cdsBit2Word/5
  In6/1 -> cdsBit2Word/6
  In7/1 -> cdsBit2Word/7
  In8/1 -> cdsBit2Word/8
  In9/1 -> cdsBit2Word/9
  In10/1 -> cdsBit2Word/10
  Sum/1 -> Out1/1
  In11/1 -> cdsBit2Word/11
  In12/1 -> cdsBit2Word/12
  In13/1 -> cdsBit2Word/13
  In14/1 -> cdsBit2Word/14
  In15/1 -> cdsBit2Word/15
  In16/1 -> cdsBit2Word/16
  In17/1 -> cdsBit2Word1/1
  In18/1 -> cdsBit2Word1/2
  In19/1 -> cdsBit2Word1/3
  In20/1 -> cdsBit2Word1/4
  In21/1 -> cdsBit2Word1/5
  In22/1 -> cdsBit2Word1/6
  In23/1 -> cdsBit2Word1/7
  In24/1 -> cdsBit2Word1/8
  In25/1 -> cdsBit2Word1/9
  In26/1 -> cdsBit2Word1/10
  In27/1 -> cdsBit2Word1/11
  In28/1 -> cdsBit2Word1/12
  In29/1 -> cdsBit2Word1/13
  In30/1 -> cdsBit2Word1/14
  In31/1 -> cdsBit2Word1/15
  In32/1 -> cdsBit2Word1/16
